simulink library "lib_spd_estimator_nodiv"  (Simulink 7.7)
settings: Solver=ode45  StartTime=0.0  StopTime=10.0  RelTol=1e-3
undefined symbols (not defined in the file): R
settings Model: Creator=lfeng  LastModifiedBy=lfeng

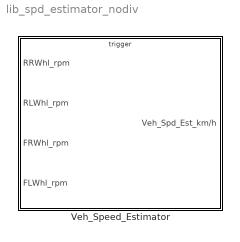
== system lib_spd_estimator_nodiv ==
  Veh_Speed_Estimator : Subsystem  TreatAsAtomicUnit=on

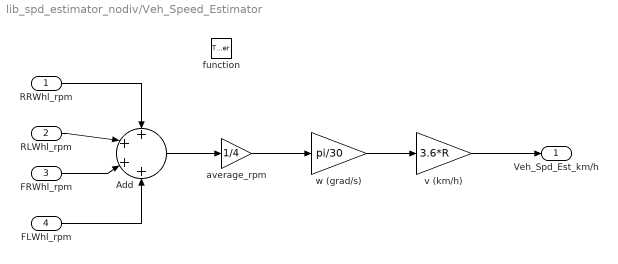
== system lib_spd_estimator_nodiv/Veh_Speed_Estimator ==
  RRWhl_rpm : Inport
  RLWhl_rpm : Inport  Port=2
  FRWhl_rpm : Inport  Port=3
  FLWhl_rpm : Inport  Port=4
  function : TriggerPort  TriggerType=function-call
  Add : Sum  Inputs=++++
  average_rpm : Gain  Gain=1/4  OutMin=0  OutMax=2000  OutDataTypeStr=double
  v (km/h) : Gain  Gain=3.6*R  OutMin=0  OutMax=200
  w (grad/s) : Gain  Gain=pi/30  OutMin=0  OutMax=250
  Veh_Spd_Est_km/h : Outport
  wires:
  RRWhl_rpm/1 -> Add/1
  RLWhl_rpm/1 -> Add/2
  FRWhl_rpm/1 -> Add/3
  FLWhl_rpm/1 -> Add/4
  Add/1 -> average_rpm/1
  w (grad/s)/1 -> v (km/h)/1
  average_rpm/1 -> w (grad/s)/1
  v (km/h)/1 -> Veh_Spd_Est_km/h/1
